simulink library "LightsLibrary"  (R2021a)
settings: Solver=VariableStepAuto  StartTime=0.0  StopTime=10.0  RelTol=1e-3
settings Model: Creator=mariekutscher  LastModifiedBy=mariekutscher

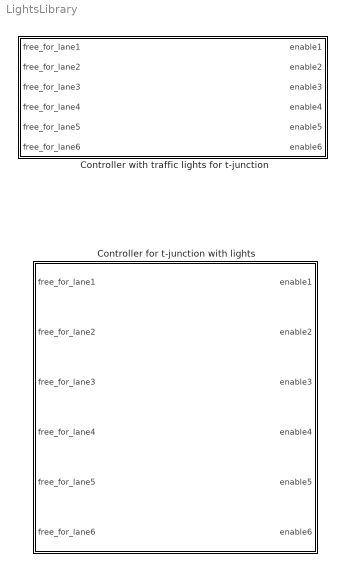
== system LightsLibrary ==
  Controller for t-junction with lights : Stateflow chart  TreatAsAtomicUnit=on  mask{green_time=10}
      mask prompts: green_time "Time for showing green"
  Controller with traffic lights for t-junction : Subsystem

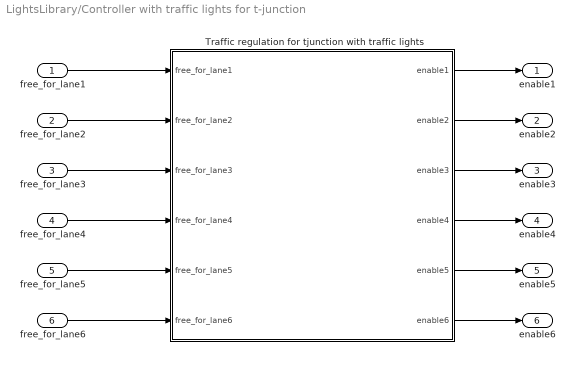
== system LightsLibrary/Controller with traffic lights for t-junction ==
  free_for_lane1 : Inport
  free_for_lane2 : Inport  Port=2
  free_for_lane3 : Inport  Port=3
  free_for_lane4 : Inport  Port=4
  free_for_lane5 : Inport  Port=5
  free_for_lane6 : Inport  Port=6
  Traffic regulation for tjunction with traffic lights : Stateflow chart  TreatAsAtomicUnit=on
  enable1 : Outport
  enable2 : Outport  Port=2
  enable3 : Outport  Port=3
  enable4 : Outport  Port=4
  enable5 : Outport  Port=5
  enable6 : Outport  Port=6
  wires:
  free_for_lane1/1 -> Traffic regulation for tjunction with traffic lights/1(free_for_lane1)
  free_for_lane2/1 -> Traffic regulation for tjunction with traffic lights/2(free_for_lane2)
  free_for_lane3/1 -> Traffic regulation for tjunction with traffic lights/3(free_for_lane3)
  free_for_lane4/1 -> Traffic regulation for tjunction with traffic lights/4(free_for_lane4)
  free_for_lane5/1 -> Traffic regulation for tjunction with traffic lights/5(free_for_lane5)
  free_for_lane6/1 -> Traffic regulation for tjunction with traffic lights/6(free_for_lane6)
  Traffic regulation for tjunction with traffic lights/1(enable1) -> enable1/1
  Traffic regulation for tjunction with traffic lights/2(enable2) -> enable2/1
  Traffic regulation for tjunction with traffic lights/3(enable3) -> enable3/1
  Traffic regulation for tjunction with traffic lights/4(enable4) -> enable4/1
  Traffic regulation for tjunction with traffic lights/5(enable5) -> enable5/1
  Traffic regulation for tjunction with traffic lights/6(enable6) -> enable6/1

== stateflow chart LightsLibrary/Controller for t-junction with lights ==
  state Enable1_3_5
    entry: enable2 = false; enable4 = false; enable6 = false;
    enable1 = true;
    enable3 = true;
    enable5 = true;
    exit: enable1 = false; enable3 = false; enable5 = false;
  state Enable1_3
    entry: enable2 = false; enable4 = false; enable5 = false; enable6 = false;
    enable1 = true;
    enable3 = true;
    exit: enable1 = false; enable3 = false;
  state Enable1_5
    entry: enable2 = false; enable3; enable4 = false; enable6 = false;
    enable1 = true;
    enable5 = true;
    exit: enable1 = false; enable5 = false;
  state Lane_1_6
    entry: enable2 = false; enable3 = false; enable4 = false; enable5 = false;
    enable1 = true;
    enable6 = true;
    exit: enable1 = false; enable6 = false;
  state Enable3_5
    entry: enable1 = false; enable2 = false; enable4 = false; enable6 = false;
    enable3 = true;
    enable5 = true;
    exit: enable3 = false; enable5 = false;
  state Lane1
    entry: enable2 = false; enable3 = false; enable4 = false; enable5 = false; enable6 = false;
    enable1 = true;
    exit: enable1 = false;
  state Lane1_3_5
  state Lane1_6
  state Lane6
    entry: enable1 = false; enable2 = false; enable3 = false; enable4 = false; enable5 = false;
    enable6 = true;
    exit: enable6 = false;
  state Enable1
    entry: enable2 = false; enable3 = false; enable4 = false;  enable5 = false; enable6 = false;
    enable1 = true;
    exit: enable1 = false;
  state Enable3
    entry: enable1 = false; enable2 = false; enable4 = false; enable5 = false; enable6 = false;
    enable3 = true;
    exit: enable3 = false;
  state Enable5
    entry: enable1 = false; enable2 = false; enable3 = false; enable4 = false; enable6 = false;
    enable5 = true;
    exit: enable5 = false;
  note: ?
  state Lane3
    entry: enable1 = false; enable2 = false; enable4 = false; enable5 = false; enable6 = false;
    enable3 = true;
    exit: enable3 = false;
  state Lane4
    entry: enable1 = false; enable2 = false; enable3 = false; enable5 = false; enable6 = false;
    enable4 = true;
    exit: enable4 = false;
  state Lane5
    entry: enable1 = false; enable2 = false; enable3 = false; enable4 = false; enable6 = false;
    enable5 = true;
    exit: enable5 = false;
  state Lane_3_4_5
  state Lane_1_2_3
  state Lane3_state123
    entry: enable2 = false; enable4 = false; enable5 = false; enable6 = false;
    enable1 = true;
    enable3 = true;
    exit: enable1 = false; enable3 = false;
  state Lane4_5
    entry: enable1 = false; enable2 = false; enable3 = false; enable6 = false;
    enable4 = true;
    enable5 = true;
    exit: enable4 = false; enable5 = false;
  state Lane2
    entry: enable2 = false; enable4 = false; enable5 = false; enable6 = false;
    enable1 = true;
    enable3 = true;
    exit: enable1 = false; enable3 = false;
  state Lane1_2_3
    entry: enable4 = false; enable5 = false; enable6 = false;
    enable1 = true;
    enable2 = true;
    enable3 = true;
    exit: enable1 = false; enable2 = false; enable3 = false;
  state Lane1_state123
    entry: enable2 = false; enable4 = false; enable5 = false; enable6 = false;
    enable1 = true;
    enable3 = true;
    exit: enable1 = false; enable3 = false;
  state Lane1_2
    entry: enable3 = false; enable4 = false; enable5 = false; enable6 = false;
    enable1 = true;
    enable2 = true;
    exit: enable1 = false; enable2 = false;
  state Lane2_3
    entry: enable1 = false; enable4 = false; enable5 = false; enable6 = false;
    enable2 = true;
    enable3 = true;
    exit: enable2 = false; enable3 = false;
  state Lane3_5
    entry: enable1 = false; enable2 = false; enable4 = false; enable6 = false;
    enable3 = true;
    enable5 = true;
    exit: enable3 = false; enable5 = false;
  state Lane1_3
    entry: enable2 = false; enable4 = false; enable5 = false; enable6 = false;
    enable1 = true;
    enable3 = true;
    exit: enable1 = false; enable3 = false;
  state Lane3_4
    entry:  enable1 = false; enable2 = false; enable5 = false; enable6 = false;
    enable3 = true;
    enable4 = true;
    exit: enable3 = false; enable4 = false;
  state Lane3_4_5
    entry: enable1 = false; enable2 = false; enable6 = false;
    enable3 = true;
    enable4 = true;
    enable5 = true;
    exit: enable3 = false; enable4 = false; enable5 = false;
  Lane1_3_5 -> Enable1_3_5 [order 1] : [free_for_lane1 == true && ...
      |  free_for_lane3 == true && ...
      | free_for_lane5 == true]
  Enable1_3_5 -> Lane_1_2_3 : [after(green_time, sec)]
  Lane1_3_5 -> Enable1_3 [order 7] : [free_for_lane1 == true && ...
      | free_for_lane3 == true]
  Lane6 -> Lane1_3_5 : [after(green_time, sec)]
  Enable1_3 -> Lane_1_2_3 : [after(green_time, sec)]
  Lane1 -> Lane1_3_5 : [after(green_time, sec)]
  Lane1_3_5 -> Enable1_5 [order 6] : [free_for_lane1 == true && ...
      | free_for_lane5 == true]
  Enable1_5 -> Lane_1_2_3 : [after(green_time, sec)]
  Lane_1_6 -> Lane1_3_5 : [after(green_time, sec)]
  Lane1_3_5 -> Enable3_5 [order 5] : [free_for_lane3 == true && ...
      | free_for_lane5 == true]
  Lane1_6 -> Lane_1_6 [order 1] : [free_for_lane1 == true &&...
      |  free_for_lane6 == true]
  Enable3_5 -> Lane_1_2_3 : [after(green_time, sec)]
  Lane1_6 -> Lane1 [order 2] : [free_for_lane1 == true]
  (default) -> Lane1_3_5
  Lane1_6 -> (junction 217) [order 4] : [free_for_lane1 == false && ...
      | free_for_lane6 == false]
  (junction 217) -> Lane1_3_5 : [after(green_time, sec)]
  Lane1_3_5 -> Enable1 [order 4] : [free_for_lane1 == true]
  Lane1_6 -> Lane6 [order 3] : [free_for_lane6 == true]
  Lane3_4 -> Lane1_6 : [after(green_time, sec)]
  Lane1_3_5 -> Enable3 [order 3] : [free_for_lane3 == true]
  Lane3_4_5 -> Lane1_6 : [after(green_time, sec)]
  Lane1_3_5 -> Enable5 [order 2] : [free_for_lane5 == true]
  Lane4_5 -> Lane1_6 : [after(green_time, sec)]
  Lane3_5 -> Lane1_6 : [after(green_time, sec)]
  Lane5 -> Lane1_6 : [after(green_time, sec)]
  Lane4 -> Lane1_6 : [after(green_time, sec)]
  Lane3 -> Lane1_6 : [after(green_time, sec)]
  (junction 214) -> Lane1_6 : [after(green_time, sec)]
  Lane1_3_5 -> (junction 208) [order 8] : [free_for_lane1 == false && ...
      | free_for_lane3 == false && ...
      | free_for_lane5 == false]
  Enable1 -> Lane_1_2_3 : [after(green_time, sec)]
  Enable3 -> Lane_1_2_3 : [after(green_time, sec)]
  Enable5 -> Lane_1_2_3 : [after(green_time, sec)]
  Lane_3_4_5 -> (junction 214) [order 8] : [free_for_lane3 == false && ...
      | free_for_lane4 == false && ...
      | free_for_lane5 == false ]
  (junction 208) -> Lane_1_2_3 : [after(green_time, sec)]
  Lane_3_4_5 -> Lane3 [order 7] : [free_for_lane3  == true]
  Lane_1_2_3 -> (junction 211) [order 8] : [free_for_lane1 == false && ...
      | free_for_lane2 == false && ...
      | free_for_lane3 == false]
  (junction 211) -> Lane_3_4_5 : [after(green_time, sec)]
  Lane_3_4_5 -> Lane4 [order 6] : [free_for_lane4 == true]
  Lane_3_4_5 -> Lane3_4 [order 2] : [free_for_lane3 == true && ...
      |  free_for_lane4 == true]
  Lane_1_2_3 -> Lane2 [order 3] : [free_for_lane2 == true]
  Lane_1_2_3 -> Lane1_state123 [order 4] : [free_for_lane1 == true ]
  Lane3_state123 -> Lane_3_4_5 : [after(green_time, sec)]
  Lane_1_2_3 -> Lane3_state123 [order 2] : [free_for_lane3 == true]
  Lane_3_4_5 -> Lane5 [order 5] : [free_for_lane5 == true]
  Lane2 -> Lane_3_4_5 : [after(green_time, sec)]
  Lane_3_4_5 -> Lane3_5 [order 3] : [free_for_lane3 == true && ...
      |  free_for_lane5 == true]
  Lane_3_4_5 -> Lane4_5 [order 4] : [free_for_lane4 == true && ...
      |  free_for_lane5 == true]
  Lane1_2_3 -> Lane_3_4_5 : [after(green_time, sec)]
  Lane_3_4_5 -> Lane3_4_5 [order 1] : [free_for_lane3 == true && ...
      |  free_for_lane4 == true && ...
      |  free_for_lane5 == true ]
  Lane1_3 -> Lane_3_4_5 : [after(green_time, sec)]
  Lane1_2 -> Lane_3_4_5 : [after(green_time, sec)]
  Lane2_3 -> Lane_3_4_5 : [after(green_time, sec)]
  Lane1_state123 -> Lane_3_4_5 : [after(green_time, sec)]
  Lane_1_2_3 -> Lane2_3 [order 5] : [free_for_lane2 == true && ...
      |  free_for_lane3 == true]
  Lane_1_2_3 -> Lane1_3 [order 6] : [free_for_lane1 == true && ...
      |  free_for_lane3 == true]
  Lane_1_2_3 -> Lane1_2 [order 7] : [free_for_lane1 == true && ...
      |  free_for_lane2 == true]
  Lane_1_2_3 -> Lane1_2_3 [order 1] : [free_for_lane1 == true && ...
      |  free_for_lane2 == true && ...
      |  free_for_lane3 == true]
  data: enable1 output boolean size=1; enable2 output boolean size=1; enable3 output boolean size=1; enable4 output boolean size=1; enable5 output boolean size=1; enable6 output boolean size=1; free_for_lane1 input; free_for_lane2 input; free_for_lane3 input; free_for_lane4 input; free_for_lane5 input; free_for_lane6 input; green_time parameter [0 ..]

== stateflow chart LightsLibrary/Controller with traffic lights for t-junction/Traffic regulation for tjunction with traffic lights ==
  state Enable1_3_5
    entry: enable2 = false; enable4 = false; enable6 = false;
    enable1 = true;
    enable3 = true;
    enable5 = true;
    exit: enable1 = false; enable3 = false; enable5 = false;
  state Enable1_3
    entry: enable2 = false; enable4 = false; enable5 = false; enable6 = false;
    enable1 = true;
    enable3 = true;
    exit: enable1 = false; enable3 = false;
  state Enable1_5
    entry: enable2 = false; enable3; enable4 = false; enable6 = false;
    enable1 = true;
    enable5 = true;
    exit: enable1 = false; enable5 = false;
  state Lane_1_6
    entry: enable2 = false; enable3 = false; enable4 = false; enable5 = false;
    enable1 = true;
    enable6 = true;
    exit: enable1 = false; enable6 = false;
  state Enable3_5
    entry: enable1 = false; enable2 = false; enable4 = false; enable6 = false;
    enable3 = true;
    enable5 = true;
    exit: enable3 = false; enable5 = false;
  state Lane1
    entry: enable2 = false; enable3 = false; enable4 = false; enable5 = false; enable6 = false;
    enable1 = true;
    exit: enable1 = false;
  state Lane1_3_5
  state Lane1_6
  state Lane6
    entry: enable1 = false; enable2 = false; enable3 = false; enable4 = false; enable5 = false;
    enable6 = true;
    exit: enable6 = false;
  state Enable1
    entry: enable2 = false; enable3 = false; enable4 = false;  enable5 = false; enable6 = false;
    enable1 = true;
    exit: enable1 = false;
  state Enable3
    entry: enable1 = false; enable2 = false; enable4 = false; enable5 = false; enable6 = false;
    enable3 = true;
    exit: enable3 = false;
  state Enable5
    entry: enable1 = false; enable2 = false; enable3 = false; enable4 = false; enable6 = false;
    enable5 = true;
    exit: enable5 = false;
  note: ?
  state Lane3
    entry: enable1 = false; enable2 = false; enable4 = false; enable5 = false; enable6 = false;
    enable3 = true;
    exit: enable3 = false;
  state Lane4
    entry: enable1 = false; enable2 = false; enable3 = false; enable5 = false; enable6 = false;
    enable4 = true;
    exit: enable4 = false;
  state Lane5
    entry: enable1 = false; enable2 = false; enable3 = false; enable4 = false; enable6 = false;
    enable5 = true;
    exit: enable5 = false;
  state Lane_3_4_5
  state Lane_1_2_3
  state Lane3_state123
    entry: enable2 = false; enable4 = false; enable5 = false; enable6 = false;
    enable1 = true;
    enable3 = true;
    exit: enable1 = false; enable3 = false;
  state Lane4_5
    entry: enable1 = false; enable2 = false; enable3 = false; enable6 = false;
    enable4 = true;
    enable5 = true;
    exit: enable4 = false; enable5 = false;
  state Lane2
    entry: enable2 = false; enable4 = false; enable5 = false; enable6 = false;
    enable1 = true;
    enable3 = true;
    exit: enable1 = false; enable3 = false;
  state Lane1_2_3
    entry: enable4 = false; enable5 = false; enable6 = false;
    enable1 = true;
    enable2 = true;
    enable3 = true;
    exit: enable1 = false; enable2 = false; enable3 = false;
  state Lane1_state123
    entry: enable2 = false; enable4 = false; enable5 = false; enable6 = false;
    enable1 = true;
    enable3 = true;
    exit: enable1 = false; enable3 = false;
  state Lane1_2
    entry: enable3 = false; enable4 = false; enable5 = false; enable6 = false;
    enable1 = true;
    enable2 = true;
    exit: enable1 = false; enable2 = false;
  state Lane2_3
    entry: enable1 = false; enable4 = false; enable5 = false; enable6 = false;
    enable2 = true;
    enable3 = true;
    exit: enable2 = false; enable3 = false;
  state Lane3_5
    entry: enable1 = false; enable2 = false; enable4 = false; enable6 = false;
    enable3 = true;
    enable5 = true;
    exit: enable3 = false; enable5 = false;
  state Lane1_3
    entry: enable2 = false; enable4 = false; enable5 = false; enable6 = false;
    enable1 = true;
    enable3 = true;
    exit: enable1 = false; enable3 = false;
  state Lane3_4
    entry:  enable1 = false; enable2 = false; enable5 = false; enable6 = false;
    enable3 = true;
    enable4 = true;
    exit: enable3 = false; enable4 = false;
  state Lane3_4_5
    entry: enable1 = false; enable2 = false; enable6 = false;
    enable3 = true;
    enable4 = true;
    enable5 = true;
    exit: enable3 = false; enable4 = false; enable5 = false;
  Lane1_3_5 -> Enable1_3_5 [order 1] : [free_for_lane1 == true && ...
      |  free_for_lane3 == true && ...
      | free_for_lane5 == true]
  Enable1_3_5 -> Lane_1_2_3 : [after(5, sec)]
  Lane1_3_5 -> Enable1_3 [order 7] : [free_for_lane1 == true && ...
      | free_for_lane3 == true]
  Lane6 -> Lane1_3_5 : [after(5, sec)]
  Lane1 -> Lane1_3_5 : [after(5, sec)]
  Lane1_3_5 -> Enable1_5 [order 6] : [free_for_lane1 == true && ...
      | free_for_lane5 == true]
  Enable1_5 -> Lane_1_2_3 : [after(5, sec)]
  Lane_1_6 -> Lane1_3_5 : [after(5, sec)]
  Lane1_3_5 -> Enable3_5 [order 5] : [free_for_lane3 == true && ...
      | free_for_lane5 == true]
  Lane1_6 -> Lane_1_6 [order 1] : [free_for_lane1 == true &&...
      |  free_for_lane6 == true]
  Enable3_5 -> Lane_1_2_3 : [after(5, sec)]
  Lane1_6 -> Lane1 [order 2] : [free_for_lane1 == true]
  (default) -> Lane1_3_5
  Lane1_3_5 -> Enable1 [order 4] : [free_for_lane1 == true]
  Lane1_6 -> Lane6 [order 3] : [free_for_lane6 == true]
  Lane3_4 -> Lane1_6 : [after(5, sec)]
  Lane1_3_5 -> Enable3 [order 3] : [free_for_lane3 == true]
  Lane3_4_5 -> Lane1_6 : [after(5, sec)]
  Lane1_3_5 -> Enable5 [order 2] : [free_for_lane5 == true]
  Lane4_5 -> Lane1_6 : [after(5, sec)]
  Lane3_5 -> Lane1_6 : [after(5, sec)]
  Lane5 -> Lane1_6 : [after(5, sec)]
  Lane4 -> Lane1_6 : [after(5, sec)]
  Lane3 -> Lane1_6 : [after(5, sec)]
  Enable1 -> Lane_1_2_3 : [after(5, sec)]
  Enable3 -> Lane_1_2_3 : [after(5, sec)]
  Enable5 -> Lane_1_2_3 : [after(5, sec)]
  Lane_3_4_5 -> Lane3 [order 7] : [free_for_lane3  == true]
  Lane_3_4_5 -> Lane4 [order 6] : [free_for_lane4 == true]
  Lane_3_4_5 -> Lane3_4 [order 2] : [free_for_lane3 == true && ...
      |  free_for_lane4 == true]
  Lane_1_2_3 -> Lane2 [order 3] : [free_for_lane2 == true]
  Lane_1_2_3 -> Lane1_state123 [order 4] : [free_for_lane1 == true ]
  Lane3_state123 -> Lane_3_4_5 : [after(5, sec)]
  Lane_1_2_3 -> Lane3_state123 [order 2] : [free_for_lane3 == true]
  Lane_3_4_5 -> Lane5 [order 5] : [free_for_lane5 == true]
  Lane2 -> Lane_3_4_5 : [ after(5, sec)]
  Lane_3_4_5 -> Lane3_5 [order 3] : [free_for_lane3 == true && ...
      |  free_for_lane5 == true]
  Lane_3_4_5 -> Lane4_5 [order 4] : [free_for_lane4 == true && ...
      |  free_for_lane5 == true]
  Lane1_2_3 -> Lane_3_4_5 : [after(5, sec)]
  Lane_3_4_5 -> Lane3_4_5 [order 1] : [free_for_lane3 == true && ...
      |  free_for_lane4 == true && ...
      |  free_for_lane5 == true ]
  Lane1_3 -> Lane_3_4_5 : [after(5, sec)]
  Lane1_2 -> Lane_3_4_5 : [after(5, sec)]
  Lane2_3 -> Lane_3_4_5 : [after(5, sec)]
  Lane1_state123 -> Lane_3_4_5 : [after(5, sec)]
  Lane_1_2_3 -> Lane2_3 [order 5] : [free_for_lane2 == true && ...
      |  free_for_lane3 == true]
  Lane_1_2_3 -> Lane1_3 [order 6] : [free_for_lane1 == true && ...
      |  free_for_lane3 == true]
  Lane_1_2_3 -> Lane1_2 [order 7] : [free_for_lane1 == true && ...
      |  free_for_lane2 == true]
  Lane_1_2_3 -> Lane1_2_3 [order 1] : [free_for_lane1 == true && ...
      |  free_for_lane2 == true && ...
      |  free_for_lane3 == true]
  data: enable1 output boolean size=1; enable2 output boolean size=1; enable3 output boolean size=1; enable4 output boolean size=1; enable5 output boolean size=1; enable6 output boolean size=1; l5 local; l6 local; counter local; l1 local; l2 local; l4 local; l3 local; free_for_lane1 input; free_for_lane2 input; free_for_lane3 input; free_for_lane4 input; free_for_lane5 input; free_for_lane6 input
